simulink model "MOSSE_HDL_final"  (Simulink 8.3)
settings: Solver=FixedStepDiscrete  SolverMode=SingleTasking  StartTime=0.0  StopTime=30*640*360  RelTol=1e-3
InitFcn:
  | %% DSPBuilder Start
  | alt_dspbuilder_update_model(bdroot)
  | %% DSPBuilder End
  | param
StopFcn:
  | % r = rcount.Data(:,:);
  | % w = wcount.Data(:,:);
  | % d = dout.Data(:,:);
  | % ir = read.Data(:,:);
  | % iw = write.Data(:,:);
  | % z = double([ir iw d r w]');
  | %logic_analyzer
values from neighbouring files (symbols this model uses):
  Gau = [4035 -3983 3832 -3589 3269 -2890 2472 -2039 1612 -1211 854 -553 ... (4096 elements, 1x4096)]    [Gauss_coeff.mat]    (also in param.m = reshape(conj(Gau'), 1, 4096))
undefined symbols (not defined in the file or in its folder): gray, psr, source_1, source_2, State_Machine, State_Transition_Table1, window_hann
libraries: allblocks_alteradspbuilder2 x166, hdlsllib x24, hdldemolib x3, simulink x2, dspsigattribs x2, dspmtrx3 x2, visionsinks x1, visiontextngfix x1, dspvision x1
(part 4 of 4)

== stateflow chart HDL_CODER_Subsystem/Main_State_Machine/MOSSE_SM ==
  settings: executeAtInitialization=1
  state state1
    % Условия по-умолчанию
    entry:
    en_img = false;
    read_img = false;
    write_img = false;
    rst_win = true;
    enb_win = false;
    mux_fft_ifft = true;
    start_fft_ifft = false;
    enb_fft_ifft = false;
    rst_gauss = true;
    enb_gauss = false;
    mux_mult = false;
    en_m_ram_g = false;
    read_g = false;
    write_g = false;
    enb_H_ram = false;
    read_H_ram = false;
    write_H_ram = false;
    mux_H1 = false;
    mux_H2 = false;
    div_complex_aclr = true;
    enb_div_ram = false;
    read_div_ram = false;
    write_div_ram = false;
    en_r = false;
    read_r = false;
    write_r = false;
    en_ifft_res = false;
    read_ifft_res = false;
    write_ifft_res = false;
    enb_psr = false;
    comp_shift_iaclr = true;
    comp_shift_finish = false;
    mem_count_clear = true;
    mem_count_en = false;
    psr_reset = true;
    count_std_enb = false;
    ifft_res_mult = false;
    g_out_contr = false;
    to_workspace_enb = false;
    to_workspace_write = false;
  state state35
    % (1) Запись изображения 128х128 в память
    entry:
    en_img = true;
    write_img = false;
  state state2
    entry:
    write_img = true;
  state state4
    % (2) Чтение изображения 64х64 с памяти и оконное преобразование изображения
    entry:
    write_img = false;
    read_img = true;
    rst_win = false;
    enb_win = true;
    mem_count_clear = false;
    % to_workspace_enb = true;
  state state3
    entry:
    mem_count_en = true;
  state state5
    % (3) Прямое преобразование Фурье входного изображения
    entry:
    start_fft_ifft = true;
    enb_fft_ifft = true;
  state state6
    entry:
    en_img = false;
    read_img = false;
    rst_win = true;
    enb_win = false;
    start_fft_ifft = false;
    enb_fft_ifft = false;
    mem_count_clear = true;
    mem_count_en = false;
  state state7
    % (4) Получение компонент для корреляционного адаптивного фильтра (H1 и H2)
    entry:
    rst_gauss = false;
    enb_gauss = true;
    % to_workspace_enb = false;
    %to_workspace_enb = true;
  state state50
    entry:
    enb_H_ram = true;
  state state8
    entry:
    write_H_ram = true;
    %to_workspace_enb = true;
  state state9
    entry:
    rst_gauss = true;
    enb_gauss = false;
    %to_workspace_enb = false;
  state state10
    % (6) Получение значений фильтра H (H = H1/H2)
    entry:
    write_H_ram = false;
    div_complex_aclr = false;
    enb_div_ram = true;
    %to_workspace_enb = false;
  state state11
    entry:
    read_H_ram = true;
  state state12
    entry:
    read_H_ram = false;
  state state13
    entry:
    div_complex_aclr = true;
    write_div_ram = true;
    %to_workspace_enb = true;
  state state14
    entry:
    write_div_ram = false;
    div_complex_aclr = false;
    read_div_ram = true;
    %to_workspace_enb = false;
  state state48
    entry:
    read_div_ram = false;
  state state15
    entry:
    read_H_ram = true;
  state state16
    entry:
    read_H_ram = false;
  state state17
    entry:
    div_complex_aclr = true;
    write_div_ram = true;
    %to_workspace_enb = true;
  state state18
    entry:
    write_div_ram = false;
    div_complex_aclr = false;
    read_div_ram = true;
    %to_workspace_enb = false;
  state state53
    entry:
    read_div_ram = false;
  state state19
    entry:
    write_div_ram = false;
    div_complex_aclr = false;
  state state35_1
    % (7) Корреляция
    % (7_1) запись нового изображения 128х128
    entry:
    en_img = true;
    write_img = false;
    ifft_res_mult = false;
    mux_fft_ifft = true;
    % psr_reset = true;
    % enb_psr = false;
  state state20
    entry:
    write_img = true;
    div_complex_aclr = true;
    enb_H_ram = false;
  state state21
    % (7_2) чтение изображения 64х64 и оконное преобразование изображения
    entry:
    write_img = false;
    read_img = true;
    rst_win = false;
    enb_win = true;
    mem_count_clear = false;
    % to_workspace_enb = true;
  state state22
    entry:
    mem_count_en = true;
  state state23
    % (7_3) прямое преобразование Фурье входного изображения
    entry:
    start_fft_ifft = true;
    enb_fft_ifft = true;
  state state25
    entry:
    en_img = false;
    read_img = false;
    rst_win = true;
    enb_win = false;
    start_fft_ifft = false;
    enb_fft_ifft = false;
    mem_count_clear = true;
    mem_count_en = false;
  state state27
    % (7_б) поэлементное перемножение преобразования Фурье с фильтром Н (корреляция)
    entry:
    enb_div_ram = true;
    read_div_ram = true;
    mux_mult = true;
    % to_workspace_enb = false;
    %to_workspace_enb = true;
  state state28
    % (7_в) запись результатов корреляции в память R
    entry:
    en_r = true;
    write_r = true;
  state state29
    entry:
    read_div_ram = false;
    enb_div_ram = false;
    %to_workspace_enb = false;
  state state30
    entry:
    write_r = false;
    mux_fft_ifft = false;
    %to_workspace_enb = false;
  state state39
    % (7_г) чтение памяти R и обратное преобразование Фурье
    entry:
    read_r = true;
  state state31
    entry:
    start_fft_ifft = true;
    enb_fft_ifft = true;
  state state38
    entry:
    start_fft_ifft = false;
    enb_fft_ifft = false;
  state state32
    entry:
    read_r = false;
    % psr_reset = true;
    % enb_psr = false;
  state state33
    entry:
    en_ifft_res = true;
    en_r = false;
    psr_reset = true;
    enb_psr = false;
    count_std_enb = false;
  state state34
    % (8) Расчет параметра PSR
    entry:
    write_ifft_res = true;
    psr_reset = false;
    enb_psr = true;
    %to_workspace_enb = true;
  state state36
    entry:
    write_ifft_res = false;
    read_ifft_res = true;
    ifft_res_mult = true;
  state state37
    entry:
    count_std_enb = true;
  state state40
    % (9) Вычисление смещения обьекта
    entry:
    read_ifft_res = false;
    en_ifft_res = false;
    comp_shift_iaclr = false;
    mem_count_en = true;
    mux_H1 = true;
    mux_H2 = true;
    en_img = true;
    ifft_res_mult = false;
    %to_workspace_enb = false;
  state state42
    % (10) Сместить начальный адрес для памяти im_RAM
    % (10_2) чтение изображение 64х64 и оконное преобразование изображения
    entry:
    read_img = true;
    % rst_win = false;
    % enb_win = true;
    mux_fft_ifft = true;
    comp_shift_finish = true;
    mem_count_clear = false;
    %to_workspace_enb = true;
  state state24
    entry:
    mem_count_en = true;
    start_fft_ifft = true;
    enb_fft_ifft = true;
    comp_shift_finish = false;
  state state47
    % (10_3) прямое преобразование Фурье входного изображения
    entry:
    % start_fft_ifft = true;
    % enb_fft_ifft = true;
    comp_shift_finish = false;
  state state26
    %(10_4) получение компонент для корреляционного адаптивного фильтра
    entry:
    en_img = false;
    read_img = false;
    rst_win = true;
    enb_win = false;
    % start_fft_ifft = false;
    % enb_fft_ifft = false;
    mem_count_clear = true;
    mem_count_en = false;
    comp_shift_iaclr = true;
  state state43
    entry:
    rst_gauss = false;
    enb_gauss = true;
    mux_mult = false;
    en_m_ram_g = true;
    psr_reset = true;
    enb_psr = false;
    % to_workspace_enb = false;
    %to_workspace_enb = true;
  state state44
    entry:
    write_g = true;
    %to_workspace_enb = true;
  state state45
    entry:
    rst_gauss = true;
    enb_gauss = false;
    g_out_contr = true;
    %to_workspace_enb = false;
  state state46
    % (10_5) Обновление компонент фильтра H1 и H2
    entry:
    write_g = false;
    read_g = true;
    enb_H_ram = true;
    write_H_ram = false;
    % to_workspace_enb = false;
  state state49
    entry:
    read_g = false;
    read_H_ram = true;
  state state54
    entry:
    read_H_ram = false;
  state state51
    entry:
    write_H_ram = true;
    % to_workspace_enb = true;
  state state10_1
    % (10_6) Получение значиний фильтра H
    entry:
    write_H_ram = false;
    div_complex_aclr = false;
    enb_div_ram = true;
  state state11_1
    entry:
    read_H_ram = true;
  state state12_1
    entry:
    read_H_ram = false;
  state state13_1
    entry:
    div_complex_aclr = true;
    write_div_ram = true;
    %to_workspace_enb = true;
  state state14_1
    entry:
    write_div_ram = false;
    div_complex_aclr = false;
    read_div_ram = true;
    %to_workspace_enb = false;
  state state48_1
    entry:
    read_div_ram = false;
  state state15_1
    entry:
    read_H_ram = true;
  state state16_1
    entry:
    read_H_ram = false;
  state state17_1
    entry:
    div_complex_aclr = true;
    write_div_ram = true;
    %to_workspace_enb = true;
  state state18_1
    entry:
    write_div_ram = false;
    div_complex_aclr = false;
    read_div_ram = true;
    %to_workspace_enb = false;
  state state53_1
    entry:
    read_div_ram = false;
  state state19_1
    entry:
    write_div_ram = false;
    div_complex_aclr = false;
  state state20_1
    % Переход к ожиданию нового кадра
    entry:
    div_complex_aclr = true;
    enb_H_ram = false;
  state state48_1_1
    entry:
    read_div_ram = false;
  state state41
    entry:
    rst_win = false;
    enb_win = true;
  state state52
    entry:
    start_fft_ifft = false;
    enb_fft_ifft = false;
  state1 -> (junction 663) [order 2]
  (default) -> state1
  (junction 663) -> state1
  state1 -> state35 [order 1] : [enable_in == true]
      | {delay = fi(0,0,5,0);
      | count = fi(0,0,13,0);}
  state35 -> (junction 664) [order 2]
  (junction 664) -> state35
  state2 -> state35 [order 2] : [img_finish == false && enable_write == false]
  state35 -> state2 [order 1] : [enable_write == true]
  state2 -> (junction 665) [order 3]
  (junction 665) -> state2
  state2 -> state4 [order 1] : [img_finish == true && enable_write == false]
  state4 -> (junction 666) [order 2]
  (junction 666) -> state4
  state4 -> state3 [order 1]
  state3 -> (junction 667) [order 2]
  (junction 667) -> state3
  state3 -> state5 [order 1]
  state5 -> (junction 668) [order 1] : [count ~= 4093]
      | {count = fi(count + 1,numerictype(0,13,0));}
  (junction 668) -> state5
  state5 -> state6 [order 2] : {count = fi(0,numerictype(0,13,0));}
  state6 -> (junction 669) [order 2]
  (junction 669) -> state6
  state6 -> state7 [order 1] : [data_ready == true]
  state7 -> (junction 670) [order 2]
  (junction 670) -> state7
  state7 -> state50 [order 1]
  state50 -> (junction 671) [order 2]
  (junction 671) -> state50
  state50 -> state8 [order 1]
  state8 -> (junction 672) [order 2]
  (junction 672) -> state8
  state8 -> state9 [order 1] : [end_fft == true]
  state9 -> (junction 673) [order 1] : [delay ~= 1]
      | {delay = fi(delay + 1,0,5,0);}
  (junction 673) -> state9
  state9 -> state10 [order 2] : {delay = fi(0,0,5,0);}
  state10 -> (junction 674) [order 1] : [delay ~= 2]
      | {delay = fi(delay + 1,0,5,0);}
  (junction 674) -> state10
  state10 -> state11 [order 2] : {delay = fi(0,0,5,0);}
  state11 -> (junction 675) [order 2]
  (junction 675) -> state11
  state11 -> state12 [order 1]
  state12 -> (junction 676) [order 2]
  (junction 676) -> state12
  state12 -> state13 [order 1]
  state13 -> (junction 677) [order 2]
  (junction 677) -> state13
  state13 -> state14 [order 1]
  state14 -> (junction 678) [order 2]
  (junction 678) -> state14
  state14 -> state48 [order 1]
  state48 -> (junction 679) [order 1] : [delay ~= 1]
      | {delay = fi(delay + 1,0,5,0);}
  (junction 679) -> state48
  state48 -> state15 [order 2] : {delay = fi(0,0,5,0);}
  state15 -> (junction 680) [order 2]
  (junction 680) -> state15
  (junction 681) -> state15
  (junction 686) -> (junction 681)
  state15 -> state16 [order 1]
  state16 -> (junction 682) [order 2]
  (junction 682) -> state16
  state16 -> state17 [order 1]
  state17 -> (junction 683) [order 2]
  (junction 683) -> state17
  state17 -> state18 [order 1]
  state18 -> (junction 684) [order 2]
  (junction 684) -> state18
  state18 -> state53 [order 1]
  state53 -> (junction 685) [order 2]
  (junction 685) -> state53
  state53 -> state19 [order 1]
  state19 -> (junction 686) [order 1] : [count ~= 4094]
      | {count = fi(count + 1,0,13,0);}
  state19 -> state35_1 [order 2] : {count = fi(0,0,13,0);}
  state35_1 -> (junction 687) [order 2]
  (junction 687) -> state35_1
  (junction 688) -> state35_1
  (junction 706) -> (junction 688)
  state20 -> state35_1 [order 2] : [img_finish == false && enable_write == false]
  state35_1 -> state20 [order 1] : [enable_write == true]
  state20 -> (junction 689) [order 3]
  (junction 689) -> state20
  state20 -> state21 [order 1] : [img_finish == true && enable_write == false]
  (junction 690) -> state20
  state21 -> (junction 691) [order 2]
  (junction 691) -> state21
  state21 -> state22 [order 1]
  state22 -> (junction 692) [order 2]
  (junction 692) -> state22
  state22 -> state23 [order 1]
  state23 -> (junction 693) [order 1] : [count ~= 4093]
      | {count = fi(count + 1,0,13,0);}
  (junction 693) -> state23
  state23 -> state25 [order 2] : {count = fi(0,0,13,0);}
  state25 -> (junction 694) [order 2]
  (junction 694) -> state25
  state25 -> state27 [order 1] : [data_ready == true]
  state27 -> (junction 695) [order 1] : [delay ~= 1]
      | {delay = fi(delay + 1,0,5,0);}
  (junction 695) -> state27
  state27 -> state28 [order 2] : {delay = fi(0,0,5,0);}
  state28 -> (junction 696) [order 2]
  (junction 696) -> state28
  state28 -> state29 [order 1] : [end_fft == true]
  state29 -> (junction 697) [order 1] : [delay ~= 1]
      | {delay = fi(delay + 1,0,5,0);}
  (junction 697) -> state29
  state29 -> state30 [order 2] : {delay = fi(0,0,5,0);}
  state30 -> (junction 698) [order 1] : [delay ~= 10]
      | {delay = fi(delay + 1,0,5,0);}
  (junction 698) -> state30
  state30 -> state39 [order 2] : {delay = fi(0,0,5,0);}
  state39 -> (junction 699) [order 2]
  (junction 699) -> state39
  state39 -> state31 [order 1]
  state31 -> (junction 700) [order 1] : [count ~= 4093]
      | {count = fi(count + 1,0,13,0);}
  (junction 700) -> state31
  state31 -> state38 [order 2] : {count = fi(0,0,13,0);}
  state38 -> (junction 701) [order 2]
  (junction 701) -> state38
  state38 -> state32 [order 1]
  state32 -> (junction 702) [order 2]
  (junction 702) -> state32
  state32 -> state33 [order 1] : [data_ready == true]
  state33 -> (junction 703) [order 2]
  (junction 703) -> state33
  state33 -> state34 [order 1]
  state34 -> (junction 704) [order 2]
  (junction 704) -> state34
  state34 -> state36 [order 1] : [psr_mean_finish == true]
  state36 -> (junction 705) [order 2]
  (junction 705) -> state36
  state36 -> state37 [order 1]
  state37 -> (junction 706) [order 2] : [psr_finish == true && psr_check == false]
  (junction 740) -> (junction 706)
  state37 -> state40 [order 1] : [psr_finish == true && psr_check == true]
  state40 -> (junction 707) [order 2] : % {delay = fi(0,0,5,0);}
  (junction 707) -> state40
  state40 -> state41 [order 1] : % [delay ~= 1]
      | % {delay = fi(delay + 1,0,5,0);}
  state41 -> (junction 708) [order 2]
  (junction 708) -> state41
  state41 -> state42 [order 1]
  state42 -> (junction 709) [order 2]
  (junction 709) -> state42
  (junction 710) -> state42
  state42 -> state24 [order 1]
  state24 -> (junction 711) [order 2]
  (junction 711) -> state24
  (junction 712) -> state24
  state24 -> state47 [order 1]
  state47 -> (junction 713) [order 1] : [count ~= 4092]
      | {count = fi(count + 1,0,13,0);}
  (junction 713) -> state47
  state47 -> state52 [order 2] : {count = fi(0,0,13,0);}
  state52 -> (junction 714) [order 2]
  (junction 714) -> state52
  state52 -> state26 [order 1]
  state26 -> (junction 715) [order 2]
  (junction 715) -> state26
  (junction 716) -> state26
  state26 -> state43 [order 1] : [data_ready == true]
  state43 -> (junction 717) [order 1] : [delay ~= 1]
      | {delay = fi(delay + 1,0,5,0);}
  (junction 717) -> state43
  state43 -> state44 [order 2] : {delay = fi(0,0,5,0);}
  state44 -> (junction 718) [order 2]
  (junction 718) -> state44
  state44 -> state45 [order 1] : [end_fft == true]
  state45 -> (junction 719) [order 1] : [delay ~= 1]
      | {delay = fi(delay + 1,0,5,0);}
  (junction 719) -> state45
  state45 -> state46 [order 2] : {delay = fi(0,0,5,0);}
  state46 -> (junction 720) [order 2]
  (junction 720) -> state46
  (junction 721) -> state46
  (junction 724) -> (junction 721)
  state46 -> state49 [order 1]
  state49 -> (junction 722) [order 2]
  (junction 722) -> state49
  state49 -> state54 [order 1]
  state54 -> (junction 723) [order 1] : [delay ~= 1]
      | {delay = fi(delay + 1,0,5,0);}
  (junction 723) -> state54
  state54 -> state51 [order 2] : {delay = fi(0,0,5,0);}
  state51 -> (junction 724) [order 1] : [count ~= 4095]
      | {count = fi(count + 1,0,13,0);}
  state51 -> state10_1 [order 2] : {count = fi(0,0,13,0);}
  state10_1 -> (junction 725) [order 1] : [delay ~= 2]
      | {delay = fi(delay + 1,0,5,0);}
  (junction 725) -> state10_1
  state10_1 -> state11_1 [order 2] : {delay = fi(0,0,5,0);}
  state11_1 -> (junction 726) [order 2]
  (junction 726) -> state11_1
  state11_1 -> state12_1 [order 1]
  state12_1 -> (junction 727) [order 2]
  (junction 727) -> state12_1
  state12_1 -> state13_1 [order 1]
  state13_1 -> (junction 728) [order 2]
  (junction 728) -> state13_1
  state13_1 -> state14_1 [order 1]
  state14_1 -> (junction 729) [order 2]
  (junction 729) -> state14_1
  state14_1 -> state48_1 [order 1]
  state48_1 -> (junction 730) [order 2]
  (junction 730) -> state48_1
  state48_1 -> state48_1_1 [order 1]
  state48_1_1 -> (junction 731) [order 2]
  (junction 731) -> state48_1_1
  state48_1_1 -> state15_1 [order 1]
  state15_1 -> (junction 732) [order 2]
  (junction 732) -> state15_1
  (junction 733) -> state15_1
  (junction 738) -> (junction 733)
  state15_1 -> state16_1 [order 1]
  state16_1 -> (junction 734) [order 2]
  (junction 734) -> state16_1
  state16_1 -> state17_1 [order 1]
  state17_1 -> (junction 735) [order 2]
  (junction 735) -> state17_1
  state17_1 -> state18_1 [order 1]
  state18_1 -> (junction 736) [order 2]
  (junction 736) -> state18_1
  state18_1 -> state53_1 [order 1]
  state53_1 -> (junction 737) [order 2]
  (junction 737) -> state53_1
  state53_1 -> state19_1 [order 1]
  state19_1 -> (junction 738) [order 1] : [count ~= 4094]
      | {count = fi(count + 1,0,13,0);}
  state19_1 -> state20_1 [order 2] : {count = fi(0,0,13,0);}
  state20_1 -> (junction 739) [order 2]
  (junction 739) -> state20_1
  state20_1 -> (junction 740) [order 1]
  data: enable_in input boolean; enable_write input boolean; en_img output boolean; read_img output boolean; write_img output boolean; img_finish input boolean; rst_win output boolean; enb_win output boolean; delay local fixdt(0,5,0); mux_fft_ifft output boolean; start_fft_ifft output boolean; enb_fft_ifft output boolean; end_fft input boolean; data_ready input boolean; rst_gauss output boolean; enb_gauss output boolean; mux_mult output boolean; en_m_ram_g output boolean; read_g output boolean; write_g output boolean; enb_H_ram output boolean; read_H_ram output boolean; write_H_ram output boolean; mux_H2 output boolean; mux_H1 output boolean; div_complex_aclr output boolean; read_H_finish input boolean; enb_div_ram output boolean; read_div_ram output boolean; write_div_ram output boolean; count local fixdt(0,13,0); to_workspace_enb output boolean; en_r output boolean; read_r output boolean; write_r output boolean; en_ifft_res output boolean; read_ifft_res output boolean; write_ifft_res output boolean; enb_psr output boolean; comp_shift_iaclr output boolean; mem_count_clear output boolean; mem_count_en output boolean; psr_check input boolean; psr_finish input boolean; psr_mean_finish input boolean; psr_reset output boolean; ifft_res_mult output boolean; g_out_contr output boolean; to_workspace_write output boolean; comp_shift_finish output boolean; count_std_enb output boolean

== stateflow chart Source/State Transition Table ==
  state state2
    entry:
    enable_write = false;
  state state1
    entry:
    enable_write = false;
  state state3
    entry:
    enable_write = true;
  state state4
    entry:
    enable_write = false;
  state1 -> (junction 986) [order 2]
  (default) -> state1
  (junction 986) -> state1
  state1 -> state2 [order 1] : {temp = 0;
      | count = 0;}
  state2 -> (junction 987) [order 2]
  (junction 987) -> state2
  (junction 988) -> state2
  (junction 991) -> (junction 988)
  state2 -> state3 [order 1] : [address == 99541 + temp*640]
  state3 -> (junction 989) [order 1] : [count ~= 127]
      | {count = count + 1;}
  (junction 989) -> state3
  state3 -> state4 [order 2] : {temp = temp + 1;
      |  count = 0;}
  state4 -> (junction 990) [order 2] : {temp = 0;}
  (junction 990) -> state4
  state4 -> (junction 991) [order 1] : [temp ~= 128]
  data: enable_write output boolean; address input uint32; temp local double; count local double

== matlab function HDL_CODER_Subsystem/Memory_Counter_Subsys/Memory Counter ==
  data: count output fixdt(0,14,0); clear input double; en input double; dx input double; dy input double
function count  = count(clear, en, dx, dy)


result_nt = numerictype(0,14,0);
count_nt = numerictype(0,7,0);

result_fm = fimath('OverflowMode', 'saturate', 'RoundMode', 'floor');
n = fi(128, 0,8,0, result_fm);
z = fi(64, 0,7,0, result_fm);
persistent count_reg column row

if isempty(column)
    column = fi(0, count_nt, result_fm);
end

if isempty(row)
    row = fi(0, count_nt, result_fm);
end

if isempty(count_reg)
    count_reg = fi((row+dy+31)*n + (column + dx+31), result_nt, result_fm);
end

if clear
    row = fi(0, count_nt, result_fm);
    column = fi(0, count_nt, result_fm);
    count_reg = fi((row+dy+31)*n + (column + dx+31), result_nt, result_fm);
elseif en
     
     if (column == (z-1))
         if(row ~= (z-1))
             inc_r = row + fi(1, count_nt, result_fm);
             row = fi(inc_r, count_nt, result_fm);
         else row = fi(0, count_nt, result_fm);
             
         end
         column = fi(0, count_nt, result_fm);
     else
         inc_c = column + fi(1, count_nt, result_fm);
         column = fi(inc_c, count_nt, result_fm);
     end
     count_reg = fi((row+dy+31)*n + (column + dx+31), result_nt, result_fm);
end

count = count_reg;

end

== stateflow chart Video_TestBench/Write_control_subsys/Write_control_STM ==
  settings: executeAtInitialization=1
  state state2
    % Автомат управления сигналом записи кадра в память
    entry:
    x_coord = x;
    y_coord = y;
    enable_write = false;
    to_workspace_enable = false;
  state state1
    % Условия по-умолчанию
    entry:
    enable_write = false;
    x_coord = fi(0,0,10,0);
    y_coord = fi(0,0,9,0);
    frame_num = uint16(0);
    to_workspace_enable = false;
  state state3
    entry:
    enable_write = true;
  state state4
    entry:
    enable_write = false;
  state state5
    % Кадр записан
    % Обновление значений смещения
    entry:
    enable_write = false;
  state state6
    % Обновление значений координат
    entry:
    enable_write = false;
    frame_num = frame_count;
    to_workspace_enable = true;
  state1 -> (junction 1074) [order 2]
  (default) -> state1
  (junction 1074) -> state1
  state1 -> state2 [order 1] : {count = fi(0,0,8,0);
      | frame_count = uint16(0);
      | x = fi(x_init,0,10,0);
      | y = fi(y_init,0,9,0);
      | temp_x = fi(x + 128,0,10,0);
      | temp_y = fi(y + count,0,9,0);
      | Dx = int8(0);
      | Dy = int8(0);}
  state2 -> (junction 1075) [order 3]
  (junction 1075) -> state2
  (junction 1076) -> state2
  state2 -> (junction 1077) [order 2] : [comp_shift_finish == true && count == 0]
  (junction 1079) -> (junction 1076)
  (junction 1077) -> (junction 1081)
  state2 -> state3 [order 1] : [addr_x == x && addr_y == temp_y && comp_shift_finish == false]
  state3 -> (junction 1078) [order 1] : [addr_x ~= temp_x]
  (junction 1078) -> state3
  state3 -> state4 [order 2] : {count = fi(count + 1,0,8,0);
      | temp_y = fi(y + count,0,9,0);}
  state4 -> (junction 1079) [order 1] : [count ~= 128]
  (junction 1083) -> (junction 1079)
  state4 -> state5 [order 2] : {count = fi(0,0,8,0);
      | frame_count = uint16(frame_count + 1);}
  state5 -> (junction 1080) [order 2]
  (junction 1080) -> state5
  (junction 1081) -> state5
  state5 -> state6 [order 1] : {Dx = dx;
      | Dy = dy;}
  state6 -> (junction 1082) [order 2]
  (junction 1082) -> state6
  state6 -> (junction 1083) [order 1] : {x = fi(x + Dx,0,10,0);
      | y = fi(y + Dy,0,9,0);
      | temp_x = fi(x + 128,0,10,0);
      | temp_y = fi(y + count,0,9,0);}
  (junction 1084) -> state6
  data: x_coord output fixdt(0,10,0); y_coord output fixdt(0,9,0); addr_x input fixdt(0,10,0); count local fixdt(0,8,0); x local fixdt(0,10,0); addr_y input fixdt(0,9,0); y local fixdt(0,9,0); dx input int8; dy input int8; Dx local int8; Dy local int8; temp_x local fixdt(0,10,0); temp_y local fixdt(0,9,0); enable_write output boolean; comp_shift_finish input boolean; to_workspace_enable output boolean; x_init input uint16; y_init input uint16; frame_count local uint16; frame_num output uint16

== matlab function Video_TestBench/Transpone Counter ==
  data: X output fixdt(0,10,0); clear input boolean; en input boolean; Y output fixdt(0,9,0)
function [X, Y]  = count(clear, en)

%result_nt = numerictype(0,12,0);
col_nt = numerictype(0,10,0);
row_nt = numerictype(0,9,0);

result_fm = fimath('OverflowMode', 'saturate', 'RoundMode', 'floor');
m = fi(640, 0,10,0, result_fm);
n = fi(360, 0,9,0, result_fm);
% persistent count_reg 
persistent column row

% if isempty(count_reg)
%     count_reg = fi(0, result_nt, result_fm);
% end

if isempty(column)
    column = fi(0, col_nt, result_fm);
end

if isempty(row)
    row = fi(0, row_nt, result_fm);
end

if clear
    row = fi(0, row_nt, result_fm);
    column = fi(0, col_nt, result_fm);
    % count_reg = fi(0, result_nt, result_fm);
elseif en
     
     if (column == (m-1))
         if(row ~= (n-1))
             inc_r = row + fi(1, row_nt, result_fm);
             row = fi(inc_r, row_nt, result_fm);
         else row = fi(0, row_nt, result_fm);
             
         end
         column = fi(0, col_nt, result_fm);
     else
         inc_c = column + fi(1, col_nt, result_fm);
         column = fi(inc_c, col_nt, result_fm);
     end
     %count_reg = fi(column*n + row, result_nt, result_fm);
end

X = column;
Y = row;
% count = count_reg;

end

== stateflow chart HDL_CODER_Subsystem/SM_memory/SM_temp_G_F/Read_Write_SM1_patched_2 ==
  settings: executeAtInitialization=1
  state state2
    entry:
    we = false;
    rst_r = false;
    rst_w = false;
    enb_w = false;
    enb_r = false;
  state state1
    entry:
    we = false;
    rst_r = true;
    enb_r = false;
    rst_w = true;
  state state3
    entry:
    we = false;
    rst_r = false;
    enb_r = true;
    rst_w = false;
    enb_w = false;
  state state4
    entry:
    we = true;
    rst_w = false;
    enb_w = true;
    rst_r = false;
    enb_r = false;
  state1 -> (junction 1159) [order 2]
  (junction 1159) -> state1
  (default) -> state1
  (junction 1160) -> state1
  (junction 1165) -> (junction 1160)
  state1 -> state2 [order 1] : [en_m == true]
  state2 -> state1 [order 4] : [en_m == false]
  state2 -> (junction 1161) [order 3] : [read == false && write == false && en_m == true]
  (junction 1161) -> state2
  state2 -> state3 [order 1] : [read == true && write == false && en_m == true]
  (junction 1162) -> state2
  (junction 1167) -> (junction 1162)
  state2 -> (junction 1163) [order 2] : [read == false && write == true && en_m == true]
  (junction 1163) -> (junction 1168)
  state3 -> state2 [order 3] : [read == false && write == false && en_m == true]
  state3 -> (junction 1164) [order 1] : [read == true && en_m == true]
  (junction 1164) -> state3
  state3 -> state4 [order 2] : [read == false && write == true && en_m == true]
  state3 -> (junction 1165) [order 4] : [en_m == false]
  (junction 1169) -> (junction 1165)
  state4 -> state3 [order 2] : [read == true && write == false && en_m == true]
  state4 -> (junction 1166) [order 1] : [write == true && en_m == true]
  (junction 1166) -> state4
  state4 -> (junction 1167) [order 3] : [read == false && write == false && en_m == true]
  (junction 1168) -> state4
  state4 -> (junction 1169) [order 4] : [en_m == false]
  data: en_m input boolean; we output boolean; rst_r output boolean; enb_r output boolean; read input boolean; write input boolean; rst_w output boolean; enb_w output boolean

== stateflow chart HDL_CODER_Subsystem/FFT2D_System/R_RAM/Read_Write_SM6 ==
  settings: executeAtInitialization=1
  state state3
    entry:
    we = true;
    rst_img = false;
    enb_img = true;
  state state1
    entry:
    we = false;
    rst_img = true;
    enb_img = false;
  state state2
    entry:
    we = false;
    rst_img = false;
    enb_img = true;
  state1 -> (junction 1224) [order 3] : [en_m == true && read == false && write == false]
  (default) -> state1
  (junction 1224) -> state1
  state1 -> (junction 1225) [order 2] : [en_m == true && read == false && write == true]
  (junction 1225) -> (junction 1230)
  (junction 1226) -> state1
  (junction 1231) -> (junction 1226)
  state1 -> state2 [order 1] : [en_m == true && read == true && write == false]
  state2 -> state1 [order 3] : [read == false && write == false]
  state2 -> (junction 1227) [order 1] : [read == true]
  (junction 1227) -> state2
  (junction 1228) -> state2
  state2 -> state3 [order 2] : [read == false && write == true]
  state3 -> state2 [order 2] : [read == true && write == false]
  state3 -> (junction 1229) [order 1] : [write == true]
  (junction 1229) -> state3
  (junction 1230) -> state3
  state3 -> (junction 1231) [order 3] : [read == false && write == false]
  data: en_m input boolean; we output boolean; rst_img output boolean; enb_img output boolean; read input boolean; write input boolean

== stateflow chart HDL_CODER_Subsystem/SM_memory/SM_RAM_IFFT/Read_Write_SM7 ==
  settings: executeAtInitialization=1
  state state3
    entry:
    we = true;
    rst_img = false;
    enb_img = true;
  state state1
    entry:
    we = false;
    rst_img = true;
    enb_img = false;
  state state2
    entry:
    we = false;
    rst_img = false;
    enb_img = true;
  state1 -> (junction 1278) [order 3] : [en_m == true && read == false && write == false]
  (default) -> state1
  (junction 1278) -> state1
  state1 -> (junction 1279) [order 2] : [en_m == true && read == false && write == true]
  (junction 1279) -> (junction 1284)
  (junction 1280) -> state1
  (junction 1285) -> (junction 1280)
  state1 -> state2 [order 1] : [en_m == true && read == true && write == false]
  state2 -> state1 [order 3] : [read == false && write == false]
  state2 -> (junction 1281) [order 1] : [read == true]
  (junction 1281) -> state2
  (junction 1282) -> state2
  state2 -> state3 [order 2] : [read == false && write == true]
  state3 -> state2 [order 2] : [read == true && write == false]
  state3 -> (junction 1283) [order 1] : [write == true]
  (junction 1283) -> state3
  (junction 1284) -> state3
  state3 -> (junction 1285) [order 3] : [read == false && write == false]
  data: en_m input boolean; we output boolean; rst_img output boolean; enb_img output boolean; read input boolean; write input boolean

== stateflow chart HDL_CODER_Subsystem/SM_memory/im_RAM_STM/Read_Write_patched_2 ==
  settings: executeAtInitialization=1
  state state2
    entry:
    we = false;
    rst_r = false;
    rst_w = false;
    enb_w = false;
    enb_r = false;
  state state1
    entry:
    we = false;
    rst_r = true;
    enb_r = false;
    rst_w = true;
  state state3
    entry:
    we = false;
    rst_r = false;
    enb_r = true;
    rst_w = false;
    enb_w = false;
  state state4
    entry:
    we = true;
    rst_w = false;
    enb_w = true;
    rst_r = false;
    enb_r = false;
  state1 -> (junction 1344) [order 2]
  (junction 1344) -> state1
  (default) -> state1
  (junction 1345) -> state1
  (junction 1350) -> (junction 1345)
  state1 -> state2 [order 1] : [en_m == true]
  state2 -> state1 [order 4] : [en_m == false]
  state2 -> (junction 1346) [order 3] : [read == false && write == false && en_m == true]
  (junction 1346) -> state2
  state2 -> state3 [order 1] : [read == true && write == false && en_m == true]
  (junction 1347) -> state2
  (junction 1352) -> (junction 1347)
  state2 -> (junction 1348) [order 2] : [read == false && write == true && en_m == true]
  (junction 1348) -> (junction 1353)
  state3 -> state2 [order 3] : [read == false && write == false && en_m == true]
  state3 -> (junction 1349) [order 1] : [read == true && en_m == true]
  (junction 1349) -> state3
  state3 -> state4 [order 2] : [read == false && write == true && en_m == true]
  state3 -> (junction 1350) [order 4] : [en_m == false]
  (junction 1354) -> (junction 1350)
  state4 -> state3 [order 2] : [read == true && write == false && en_m == true]
  state4 -> (junction 1351) [order 1] : [write == true && en_m == true]
  (junction 1351) -> state4
  state4 -> (junction 1352) [order 3] : [read == false && write == false && en_m == true]
  (junction 1353) -> state4
  state4 -> (junction 1354) [order 4] : [en_m == false]
  data: en_m input boolean; we output boolean; rst_r output boolean; enb_r output boolean; read input boolean; write input boolean; rst_w output boolean; enb_w output boolean

== stateflow chart HDL_CODER_Subsystem/SM_memory/SM_memory_H1_H2/Read_Write_SM1_patched_1 ==
  settings: executeAtInitialization=1
  state state2
    entry:
    we = false;
    rst_r = false;
    rst_w = false;
    enb_w = false;
    enb_r = false;
  state state1
    entry:
    we = false;
    rst_r = true;
    enb_r = false;
    rst_w = true;
  state state3
    entry:
    we = false;
    rst_r = false;
    enb_r = true;
    rst_w = false;
    enb_w = false;
  state state4
    entry:
    we = true;
    rst_w = false;
    enb_w = true;
    rst_r = false;
    enb_r = false;
  state1 -> (junction 1421) [order 2]
  (junction 1421) -> state1
  (default) -> state1
  (junction 1422) -> state1
  (junction 1427) -> (junction 1422)
  state1 -> state2 [order 1] : [en_m == true]
  state2 -> state1 [order 4] : [en_m == false]
  state2 -> (junction 1423) [order 3] : [read == false && write == false && en_m == true]
  (junction 1423) -> state2
  state2 -> state3 [order 1] : [read == true && write == false && en_m == true]
  (junction 1424) -> state2
  (junction 1429) -> (junction 1424)
  state2 -> (junction 1425) [order 2] : [read == false && write == true && en_m == true]
  (junction 1425) -> (junction 1430)
  state3 -> state2 [order 3] : [read == false && write == false && en_m == true]
  state3 -> (junction 1426) [order 1] : [read == true && en_m == true]
  (junction 1426) -> state3
  state3 -> state4 [order 2] : [read == false && write == true && en_m == true]
  state3 -> (junction 1427) [order 4] : [en_m == false]
  (junction 1431) -> (junction 1427)
  state4 -> state3 [order 2] : [read == true && write == false && en_m == true]
  state4 -> (junction 1428) [order 1] : [write == true && en_m == true]
  (junction 1428) -> state4
  state4 -> (junction 1429) [order 3] : [read == false && write == false && en_m == true]
  (junction 1430) -> state4
  state4 -> (junction 1431) [order 4] : [en_m == false]
  data: en_m input boolean; we output boolean; rst_r output boolean; enb_r output boolean; read input boolean; write input boolean; rst_w output boolean; enb_w output boolean

== stateflow chart HDL_CODER_Subsystem/SM_memory/SM_RAM_IFFT_res/Read_Write_SM1_patched_2 ==
  settings: executeAtInitialization=1
  state state2
    entry:
    we = false;
    rst_r = false;
    rst_w = false;
    enb_w = false;
    enb_r = false;
  state state1
    entry:
    we = false;
    rst_r = true;
    enb_r = false;
    rst_w = true;
  state state3
    entry:
    we = false;
    rst_r = false;
    enb_r = true;
    rst_w = false;
    enb_w = false;
  state state4
    entry:
    we = true;
    rst_w = false;
    enb_w = true;
    rst_r = false;
    enb_r = false;
  state1 -> (junction 1498) [order 2]
  (junction 1498) -> state1
  (default) -> state1
  (junction 1499) -> state1
  (junction 1504) -> (junction 1499)
  state1 -> state2 [order 1] : [en_m == true]
  state2 -> state1 [order 4] : [en_m == false]
  state2 -> (junction 1500) [order 3] : [read == false && write == false && en_m == true]
  (junction 1500) -> state2
  state2 -> state3 [order 1] : [read == true && write == false && en_m == true]
  (junction 1501) -> state2
  (junction 1506) -> (junction 1501)
  state2 -> (junction 1502) [order 2] : [read == false && write == true && en_m == true]
  (junction 1502) -> (junction 1507)
  state3 -> state2 [order 3] : [read == false && write == false && en_m == true]
  state3 -> (junction 1503) [order 1] : [read == true && en_m == true]
  (junction 1503) -> state3
  state3 -> state4 [order 2] : [read == false && write == true && en_m == true]
  state3 -> (junction 1504) [order 4] : [en_m == false]
  (junction 1508) -> (junction 1504)
  state4 -> state3 [order 2] : [read == true && write == false && en_m == true]
  state4 -> (junction 1505) [order 1] : [write == true && en_m == true]
  (junction 1505) -> state4
  state4 -> (junction 1506) [order 3] : [read == false && write == false && en_m == true]
  (junction 1507) -> state4
  state4 -> (junction 1508) [order 4] : [en_m == false]
  data: en_m input boolean; we output boolean; rst_r output boolean; enb_r output boolean; read input boolean; write input boolean; rst_w output boolean; enb_w output boolean

== matlab function HDL_CODER_Subsystem/Comp_Shift_code_Subsys/Comp_Shift_code ==
  data: iaclr input double; max_num input double; dx output double; dy output double
function [dx, dy]  = count(iaclr, max_num)

numtype_nt = numerictype(1,8,0);

numtype_fm = fimath('OverflowMode', 'saturate', 'RoundMode', 'zero');
dim = fi(64, 0,8,0, numtype_fm);
persistent Dx Dy q r

if isempty(Dx)
    Dx = fi(0, numtype_nt, numtype_fm);
end

if isempty(Dy)
    Dy = fi(0, numtype_nt, numtype_fm);
end

if isempty(q)
    q = fi(0, numtype_nt, numtype_fm);
end

if isempty(r)
    r = fi(0, numtype_nt, numtype_fm);
end

% if isempty(count_reg)
%     count_reg = fi((row+dy + 31)*n + (column + dx+31), result_nt, result_fm);
% end

if iaclr
    Dx = fi(0, numtype_nt, numtype_fm);
    Dy = fi(0, numtype_nt, numtype_fm);
    q = fi(0, numtype_nt, numtype_fm);
    r = fi(0, numtype_nt, numtype_fm);
    %count_reg = fi((row+dy + 31)*n + (column + dx+31), result_nt, result_fm);
else
    q = fi((max_num/dim), numtype_nt, numtype_fm);
    r = fi((max_num - q*dim), numtype_nt, numtype_fm);
    Dx = fi((r - 31), numtype_nt, numtype_fm);
    Dy = fi((q - 31), numtype_nt, numtype_fm);
end

dx = Dx;
dy = Dy;

end
